simulink model "sst_three_phase_dab_three_levels_inv"  (R2025b)
settings: Solver=ode23tb  StartTime=0.0  StopTime=simlength  FixedStep=tc  MaxStep=tc
values from neighbouring files (symbols this model uses):
  Adrso = eye(2) + Arso*ts_inv    [init_model.m]
  Aresd_max = eye(2) + Ares_max*ts_afe    [init_model.m]
  Aresd_min = eye(2) + Ares_min*ts_afe    [init_model.m]
  Aresd_nom = eye(2) + Ares_nom*ts_afe    [init_model.m]
  Bresd = Bres*ts_afe    [init_model.m]
  CFi_dc2 = 900e-6*4    (= 0.0036)    [init_model.m]
  Cresd = Cres    [init_model.m]
  Crso = [1 0]    [init_model.m]
  delta = 0.025    [init_model.m]
  freq = 50    [init_model.m]
  Iac_FS = I_phase_normalization_factor    [init_model.m]
  Idc_FS = max(Idab1_dc_nom,Idab2_dc_nom) * margin_factor    [init_model.m]
  iph_grid_pu_ref = 3.75    [init_model.m]
  ki_afe = 18    [init_model.m]
  ki_pll = 3140    [init_model.m]
  ki_rpi = 18    [init_model.m]
  kp_afe = 0.25    [init_model.m]
  kp_pll = 314    [init_model.m]
  kp_rpi = 0.25    [init_model.m]
  Ldrso = acker(Adrso',Crso',polesdrso)'    [init_model.m]
  LFu1_AFE = 0.33e-3    (= 0.00033)    [init_model.m]
  n_modules = 2    [init_model.m]
  RLFu1_AFE = 157*0.05*LFu1_AFE    (= 0.0025905)    [init_model.m]
  tc = ts_dab/1000*24    (= 1e-06)    [init_model.m]
  ts_afe = 1/fPWM_AFE    (= 0.00025)    [init_model.m]
  ts_inv = 1/fPWM_INV    (= 0.00025)    [init_model.m]
  Vac_FS = V_phase_normalization_factor    [init_model.m]
  Vdab2_dc_nom = 1500    [init_model.m]
  Vdc_FS = max(Vdab1_dc_nom,Vdab2_dc_nom) * margin_factor    [init_model.m]
undefined symbols (not defined in the file or in its folder): omega_grid_nom, V_phase_normalization_factor
libraries: fl_lib x80, nesl_utility x55, discrete_time_low_pass_filter x6, single_phase_transformer x6, pi_ctrl x4, three_phase_inverter_ideal_switch_based_model x4, three_phase_inverter_mosfet_based_with_thermal_model x4, single_phase_transformer_lib x3, three_phase_dab_modulator x2, dclink_for_three_levels x2, single_phase_three_levels_PWM_modulator x2, dq_vector_pi x2
(part 2 of 5)

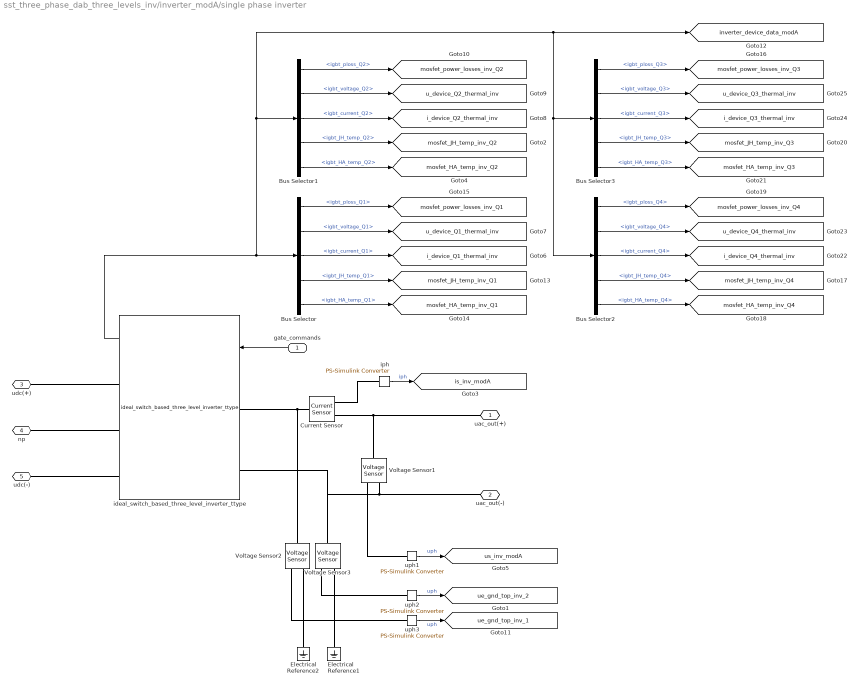
== system sst_three_phase_dab_three_levels_inv/inverter_modA/single phase inverter ==
  gate_commands : Inport
  Bus Selector : BusSelector  OutputSignals=igbt_ploss_Q1,igbt_voltage_Q1,igbt_current_Q1,igbt_JH_temp_Q1,igbt_HA_temp_Q1
  Bus Selector1 : BusSelector  OutputSignals=igbt_ploss_Q2,igbt_voltage_Q2,igbt_current_Q2,igbt_JH_temp_Q2,igbt_HA_temp_Q2
  Bus Selector2 : BusSelector  OutputSignals=igbt_ploss_Q4,igbt_voltage_Q4,igbt_current_Q4,igbt_JH_temp_Q4,igbt_HA_temp_Q4
  Bus Selector3 : BusSelector  OutputSignals=igbt_ploss_Q3,igbt_voltage_Q3,igbt_current_Q3,igbt_JH_temp_Q3,igbt_HA_temp_Q3
  Current Sensor : fl_lib/Electrical/Electrical Sensors/Current Sensor
  Electrical Reference1 : fl_lib/Electrical/Electrical Elements/Electrical Reference
  Electrical Reference2 : fl_lib/Electrical/Electrical Elements/Electrical Reference
  Voltage Sensor1 : fl_lib/Electrical/Electrical Sensors/Voltage Sensor
  Voltage Sensor2 : fl_lib/Electrical/Electrical Sensors/Voltage Sensor
  Voltage Sensor3 : fl_lib/Electrical/Electrical Sensors/Voltage Sensor
  ideal_switch_based_three_level_inverter_ttype : full_bridge_three_level_ttype_igbt_based_model/ideal_switch_based_three_level_inverter_ttype  Vth_inv_t=inv_t.Vth  Vce_sat_inv_t=inv_t.Vce_sat  Rce_on_inv_t=inv_t.Rce_on  Eon_inv_t=inv_t.Eon  Eoff_inv_t=inv_t.Eoff  Erec_inv_t=inv_t.Erec  Ion_sw_loss_inv_t=inv_t.Ion_sw_losses  Voff_sw_loss_inv_t=inv_t.Voff_sw_losses  Vdon_diode_inv_t=inv_t.Vdon_diode  Rdon_diode_inv_t=inv_t.Rdon_diode  rth_mosfet_JH_inv_t=inv_t.Rth_switch_JH  rth_mosfet_HA_inv_t=Rth_switch_HA  Csnubber_inv_t=inv_t.Csnubber  Rsnubber_inv_t=inv_t.Rsnubber  Vth_inv=inv.Vth  Vce_sat_inv=inv.Vce_sat  Rce_on_inv=inv.Rce_on  Eon_inv=inv.Eon  Eoff_inv=inv.Eoff  Erec_inv=inv.Erec  Ion_sw_loss_inv=inv.Ion_sw_losses  Voff_sw_loss_inv=inv.Voff_sw_losses  Vdon_diode_inv=inv.Vdon_diode  Rdon_diode_inv=inv.Rdon_diode  rth_mosfet_JH_inv=inv.Rth_switch_JH  rth_mosfet_HA_inv=Rth_mosfet_HA  Csnubber_inv=inv.Csnubber  Rsnubber_inv=inv.Rsnubber  tc=tc  JunctionTermalMass=JunctionTermalMass  mass_heatsink=weigth  specific_heat=cp_al  Tambient=Tambient  DThs_init=DThs_init
  iph : nesl_utility/PS-Simulink Converter  PhysicalDomain=network_engine_domain  SubClassName=ps_output  LeftPortType=input  RightPortType=output  PseudoPeriodic=off  Frequencies=[]  VectorFormat=1-D array  Unit=A  AffineConversion=off
  uph1 : nesl_utility/PS-Simulink Converter  PhysicalDomain=network_engine_domain  SubClassName=ps_output  LeftPortType=input  RightPortType=output  PseudoPeriodic=off  Frequencies=[]  VectorFormat=1-D array  Unit=V  AffineConversion=off
  uph2 : nesl_utility/PS-Simulink Converter  PhysicalDomain=network_engine_domain  SubClassName=ps_output  LeftPortType=input  RightPortType=output  PseudoPeriodic=off  Frequencies=[]  VectorFormat=1-D array  Unit=V  AffineConversion=off
  uph3 : nesl_utility/PS-Simulink Converter  PhysicalDomain=network_engine_domain  SubClassName=ps_output  LeftPortType=input  RightPortType=output  PseudoPeriodic=off  Frequencies=[]  VectorFormat=1-D array  Unit=V  AffineConversion=off
  uac_out(+) : PMIOPort  Side=Left
  uac_out(-) : PMIOPort  Port=2  Side=Left
  udc(+) : PMIOPort  Port=3  Side=Right
  np : PMIOPort  Port=4  Side=Right
  udc(-) : PMIOPort  Port=5  Side=Right
  tag scope: i_device_Q1_thermal_inv=global, i_device_Q2_thermal_inv=global, i_device_Q3_thermal_inv=global, i_device_Q4_thermal_inv=global, inverter_device_data_modA=global, is_inv_modA=global, mosfet_HA_temp_inv_Q1=global, mosfet_HA_temp_inv_Q2=global, mosfet_HA_temp_inv_Q3=global, mosfet_HA_temp_inv_Q4=global, mosfet_JH_temp_inv_Q1=global, mosfet_JH_temp_inv_Q2=global, mosfet_JH_temp_inv_Q3=global, mosfet_JH_temp_inv_Q4=global, mosfet_power_losses_inv_Q1=global, mosfet_power_losses_inv_Q2=global, mosfet_power_losses_inv_Q3=global, mosfet_power_losses_inv_Q4=global, u_device_Q1_thermal_inv=global, u_device_Q2_thermal_inv=global, u_device_Q3_thermal_inv=global, u_device_Q4_thermal_inv=global, ue_gnd_top_inv_1=global, ue_gnd_top_inv_2=global, us_inv_modA=global
  wires:
  iph/1 -> [is_inv_modA]  "iph"
  uph1/1 -> [us_inv_modA]  "uph"
  gate_commands/1 -> ideal_switch_based_three_level_inverter_ttype/1
  Bus Selector/1 -> [mosfet_power_losses_inv_Q1]  "<igbt_ploss_Q1>"
  Bus Selector/2 -> [u_device_Q1_thermal_inv]  "<igbt_voltage_Q1>"
  Bus Selector/3 -> [i_device_Q1_thermal_inv]  "<igbt_current_Q1>"
  Bus Selector/4 -> [mosfet_JH_temp_inv_Q1]  "<igbt_JH_temp_Q1>"
  Bus Selector/5 -> [mosfet_HA_temp_inv_Q1]  "<igbt_HA_temp_Q1>"
  Bus Selector1/4 -> [mosfet_JH_temp_inv_Q2]  "<igbt_JH_temp_Q2>"
  Bus Selector1/5 -> [mosfet_HA_temp_inv_Q2]  "<igbt_HA_temp_Q2>"
  Bus Selector1/3 -> [i_device_Q2_thermal_inv]  "<igbt_current_Q2>"
  Bus Selector1/2 -> [u_device_Q2_thermal_inv]  "<igbt_voltage_Q2>"
  Bus Selector1/1 -> [mosfet_power_losses_inv_Q2]  "<igbt_ploss_Q2>"
  uph2/1 -> [ue_gnd_top_inv_2]  "uph"
  uph3/1 -> [ue_gnd_top_inv_1]  "uph"
  ideal_switch_based_three_level_inverter_ttype/1 -> Bus Selector2/1, Bus Selector3/1, [inverter_device_data_modA], Bus Selector1/1, Bus Selector/1
  Bus Selector3/1 -> [mosfet_power_losses_inv_Q3]  "<igbt_ploss_Q3>"
  Bus Selector3/2 -> [u_device_Q3_thermal_inv]  "<igbt_voltage_Q3>"
  Bus Selector3/3 -> [i_device_Q3_thermal_inv]  "<igbt_current_Q3>"
  Bus Selector3/5 -> [mosfet_HA_temp_inv_Q3]  "<igbt_HA_temp_Q3>"
  Bus Selector3/4 -> [mosfet_JH_temp_inv_Q3]  "<igbt_JH_temp_Q3>"
  Bus Selector2/5 -> [mosfet_HA_temp_inv_Q4]  "<igbt_HA_temp_Q4>"
  Bus Selector2/4 -> [mosfet_JH_temp_inv_Q4]  "<igbt_JH_temp_Q4>"
  Bus Selector2/3 -> [i_device_Q4_thermal_inv]  "<igbt_current_Q4>"
  Bus Selector2/2 -> [u_device_Q4_thermal_inv]  "<igbt_voltage_Q4>"
  Bus Selector2/1 -> [mosfet_power_losses_inv_Q4]  "<igbt_ploss_Q4>"
  connections:
  Current Sensor/RConn1 -- iph/LConn1
  Current Sensor/RConn2 -- Voltage Sensor1/LConn1 -- uac_out(+)/RConn1
  Voltage Sensor1/RConn1 -- uph1/LConn1
  Voltage Sensor1/RConn2 -- ideal_switch_based_three_level_inverter_ttype/LConn2 -- Voltage Sensor3/LConn1 -- uac_out(-)/RConn1
  ideal_switch_based_three_level_inverter_ttype/RConn1 -- udc(+)/RConn1
  Current Sensor/LConn1 -- ideal_switch_based_three_level_inverter_ttype/LConn1 -- Voltage Sensor2/LConn1
  ideal_switch_based_three_level_inverter_ttype/RConn3 -- udc(-)/RConn1
  Electrical Reference2/LConn1 -- Voltage Sensor2/RConn2
  Electrical Reference1/LConn1 -- Voltage Sensor3/RConn2
  uph2/LConn1 -- Voltage Sensor3/RConn1
  uph3/LConn1 -- Voltage Sensor2/RConn1
  np/RConn1 -- ideal_switch_based_three_level_inverter_ttype/RConn2

== system sst_three_phase_dab_three_levels_inv/inverter_modA/single phase inverter control1 ==
  Constant : Constant
  acquisition_and_scaling_current : Subsystem
  acquisition_and_scaling_dc_voltage : Subsystem
  acquisition_and_scaling_voltage : Subsystem
  acquisition_and_scaling_voltage1 : Subsystem
  inverter_current_output_pu_reference : Subsystem
  pwm modulator : Subsystem
  rpi_based_single_phase_inverter_ctrl : Subsystem
  gate_cmds : Outport
  u_ctrl_out : Outport  Port=2
  tag scope: phase_synch_modA=global
  wires:
  [is_inv_modA] -> acquisition_and_scaling_current/1(in)
  pwm modulator/1(gate_cmds) -> gate_cmds/1
  [TRGO_INV_1] -> rpi_based_single_phase_inverter_ctrl/Trigger
  [inverter_voltage_output_modA] -> acquisition_and_scaling_voltage/1(in)
  acquisition_and_scaling_current/1(out) -> rpi_based_single_phase_inverter_ctrl/2(is_inv_pu)  "is_inv_pu"
  acquisition_and_scaling_voltage/1(out) -> rpi_based_single_phase_inverter_ctrl/1(inverter_voltage_output_pu)  "inverter_voltage_output_pu"
  inverter_current_output_pu_reference/1(inverter_current_output_pu_reference) -> rpi_based_single_phase_inverter_ctrl/3(is_inv_pu_reference)  "inverter_current_output_pu_reference"
  [dclink_voltage_inverter_modA] -> acquisition_and_scaling_dc_voltage/1(in)
  rpi_based_single_phase_inverter_ctrl/1(u_ctrl_out) -> u_ctrl_out/1, pwm modulator/1(vout)
  acquisition_and_scaling_voltage1/1(out) -> rpi_based_single_phase_inverter_ctrl/5(u_line_pu)  "ac_grid_voltage_pu"
  [ac_grid_voltage] -> acquisition_and_scaling_voltage1/1(in)
  rpi_based_single_phase_inverter_ctrl/2(phase_grid_modA) -> [phase_synch_modA]
  Constant/1 -> rpi_based_single_phase_inverter_ctrl/4(dclink_voltage_pu)
  [time_afe_module_1] -> rpi_based_single_phase_inverter_ctrl/6(time_afe_module_1)  "time_afe_module_1"

== system sst_three_phase_dab_three_levels_inv/inverter_modB/single phase inverter ==
  gate_commands : Inport
  Bus Selector : BusSelector  OutputSignals=switch_voltage_Q1,switch_current_Q1
  Current Sensor : fl_lib/Electrical/Electrical Sensors/Current Sensor
  Electrical Reference1 : fl_lib/Electrical/Electrical Elements/Electrical Reference
  Electrical Reference2 : fl_lib/Electrical/Electrical Elements/Electrical Reference
  Voltage Sensor1 : fl_lib/Electrical/Electrical Sensors/Voltage Sensor
  Voltage Sensor2 : fl_lib/Electrical/Electrical Sensors/Voltage Sensor
  Voltage Sensor3 : fl_lib/Electrical/Electrical Sensors/Voltage Sensor
  ideal_switch_based_three_level_inverter_ttype : full_bridge_three_level_ttype_ideal_switch_based_model/ideal_switch_based_three_level_inverter_ttype  Vth=5.5  Ron=1.5e-3  Vdon_diode=2  Rdon_diode=0.15e-3  Csnubber=10e-9  Rsnubber=2200
  iph : nesl_utility/PS-Simulink Converter  PhysicalDomain=network_engine_domain  SubClassName=ps_output  LeftPortType=input  RightPortType=output  PseudoPeriodic=off  Frequencies=[]  VectorFormat=1-D array  Unit=A  AffineConversion=off
  uph1 : nesl_utility/PS-Simulink Converter  PhysicalDomain=network_engine_domain  SubClassName=ps_output  LeftPortType=input  RightPortType=output  PseudoPeriodic=off  Frequencies=[]  VectorFormat=1-D array  Unit=V  AffineConversion=off
  uph2 : nesl_utility/PS-Simulink Converter  PhysicalDomain=network_engine_domain  SubClassName=ps_output  LeftPortType=input  RightPortType=output  PseudoPeriodic=off  Frequencies=[]  VectorFormat=1-D array  Unit=V  AffineConversion=off
  uph3 : nesl_utility/PS-Simulink Converter  PhysicalDomain=network_engine_domain  SubClassName=ps_output  LeftPortType=input  RightPortType=output  PseudoPeriodic=off  Frequencies=[]  VectorFormat=1-D array  Unit=V  AffineConversion=off
  uac_out(+) : PMIOPort  Side=Left
  uac_out(-) : PMIOPort  Port=2  Side=Left
  udc(+) : PMIOPort  Port=3  Side=Right
  np : PMIOPort  Port=4  Side=Right
  udc(-) : PMIOPort  Port=5  Side=Right
  tag scope: i_device_Q1_ideal_inv_modB=global, inverter_device_data_modB=global, is_inv_modB=global, u_device_Q1_ideal_inv_modB=global, ue_gnd_bottom_inv_1=global, ue_gnd_bottom_inv_2=global, us_inv_modB=global
  wires:
  gate_commands/1 -> ideal_switch_based_three_level_inverter_ttype/1
  uph1/1 -> [us_inv_modB]  "uph"
  iph/1 -> [is_inv_modB]  "iph"
  uph3/1 -> [ue_gnd_bottom_inv_1]  "uph"
  uph2/1 -> [ue_gnd_bottom_inv_2]  "uph"
  ideal_switch_based_three_level_inverter_ttype/1 -> [inverter_device_data_modB], Bus Selector/1
  Bus Selector/2 -> [i_device_Q1_ideal_inv_modB]  "<switch_current_Q1>"
  Bus Selector/1 -> [u_device_Q1_ideal_inv_modB]  "<switch_voltage_Q1>"
  connections:
  ideal_switch_based_three_level_inverter_ttype/RConn3 -- udc(-)/RConn1
  Voltage Sensor2/LConn1 -- ideal_switch_based_three_level_inverter_ttype/LConn1 -- Current Sensor/LConn1
  ideal_switch_based_three_level_inverter_ttype/RConn1 -- udc(+)/RConn1
  uac_out(-)/RConn1 -- ideal_switch_based_three_level_inverter_ttype/LConn2 -- Voltage Sensor3/LConn1 -- Voltage Sensor1/RConn2
  Voltage Sensor1/RConn1 -- uph1/LConn1
  uac_out(+)/RConn1 -- Voltage Sensor1/LConn1 -- Current Sensor/RConn2
  Current Sensor/RConn1 -- iph/LConn1
  Electrical Reference2/LConn1 -- Voltage Sensor2/RConn2
  uph2/LConn1 -- Voltage Sensor3/RConn1
  uph3/LConn1 -- Voltage Sensor2/RConn1
  Electrical Reference1/LConn1 -- Voltage Sensor3/RConn2
  np/RConn1 -- ideal_switch_based_three_level_inverter_ttype/RConn2

== system sst_three_phase_dab_three_levels_inv/inverter_modB/single phase inverter control1 ==
  Constant : Constant
  acquisition_and_scaling_current : Subsystem
  acquisition_and_scaling_dc_voltage : Subsystem
  acquisition_and_scaling_voltage : Subsystem
  acquisition_and_scaling_voltage1 : Subsystem
  inverter_current_output_pu_reference : Subsystem
  pwm modulator : Subsystem
  rpi_based_single_phase_inverter_ctrl : Subsystem
  gate_cmds : Outport
  tag scope: phase_synch_modB=global
  wires:
  pwm modulator/1(gate_cmds) -> gate_cmds/1
  rpi_based_single_phase_inverter_ctrl/2(phase_grid_modA) -> [phase_synch_modB]
  rpi_based_single_phase_inverter_ctrl/1(u_ctrl_out) -> pwm modulator/1(vout)
  [u_ctrl_out_master] -> rpi_based_single_phase_inverter_ctrl/6(u_ctrl_out_master)  "u_ctrl_out_master"
  Constant/1 -> rpi_based_single_phase_inverter_ctrl/4(dclink_voltage_pu)
  acquisition_and_scaling_voltage1/1(out) -> rpi_based_single_phase_inverter_ctrl/5(u_line_pu)  "u_line_pu"
  acquisition_and_scaling_current/1(out) -> rpi_based_single_phase_inverter_ctrl/2(is_inv_pu)  "is_inv_pu"
  [inverter_voltage_output_modB] -> acquisition_and_scaling_voltage/1(in)
  [ac_grid_voltage] -> acquisition_and_scaling_voltage1/1(in)
  acquisition_and_scaling_voltage/1(out) -> rpi_based_single_phase_inverter_ctrl/1(inverter_voltage_output_pu)  "inverter_voltage_output_pu"
  [dclink_voltage_inverter_modB] -> acquisition_and_scaling_dc_voltage/1(in)
  [is_inv_modB] -> acquisition_and_scaling_current/1(in)
  inverter_current_output_pu_reference/1(inverter_current_output_pu_reference) -> rpi_based_single_phase_inverter_ctrl/3(is_inv_pu_reference)  "inverter_current_output_pu_reference"
  [TRGO_INV_2] -> rpi_based_single_phase_inverter_ctrl/Trigger

== system sst_three_phase_dab_three_levels_inv/line_source/phase_gen ==
  Constant4 : Constant  Value=50*2*pi
  Integrator : Integrator
  bounder1 : MATLAB Function  TreatAsAtomicUnit=on
  phase_gen : Outport  VectorParamsAs1DForOutWhenUnconnected=off
  wires:
  Constant4/1 -> Integrator/1
  Integrator/1 -> bounder1/1(u)
  bounder1/1(y) -> phase_gen/1  "grid_emu_phase"

== system sst_three_phase_dab_three_levels_inv/scopes/scopes_dab_modA ==
  Bus Selector : BusSelector  OutputSignals=mosfet_ploss_Q1,mosfet_ploss_Q2
  Bus Selector1 : BusSelector  OutputSignals=mosfet_ploss_Q1,mosfet_ploss_Q2
  dab TR i2/i1 modA : Scope  NumInputPorts=2
      settings: SampleTime=tc  ActiveDisplayYMinimum=-1515.8601129634949  ActiveDisplayYMaximum=1519.4045908602914  DataLoggingVariableName=ScopeData13
  dab TR u2/u1 modA : Scope  NumInputPorts=2
      settings: SampleTime=tc  ActiveDisplayYMinimum=-893.62031856834165  ActiveDisplayYMaximum=653.92363611228757  DataLoggingVariableName=ScopeData4
  dab current output/input modA : Scope  NumInputPorts=2
      settings: SampleTime=tc  ActiveDisplayYMinimum=-34.407086049322743  ActiveDisplayYMaximum=284.20809963586862  DataLoggingVariableName=ScopeData8
  dab outputs modA : Scope  NumInputPorts=2
      settings: SampleTime=tc  ActiveDisplayYMinimum=-1504.2584903012705  ActiveDisplayYMaximum=905.23681286440785  DataLoggingVariableName=ScopeData6
  dab voltage input/output modA : Scope  NumInputPorts=2
      settings: SampleTime=tc  ActiveDisplayYMinimum=-224.45374462345234  ActiveDisplayYMaximum=1977.0471198962268  DataLoggingVariableName=ScopeData10
  dab_analysis_modA : Scope  NumInputPorts=4
      settings: SampleTime=tc  ActiveDisplayYMinimum=-2404.4721774395748  ActiveDisplayYMaximum=2406.0057347567245  DataLoggingVariableName=ScopeData15
  dab_analysis_power loss : Scope  NumInputPorts=4
      settings: SampleTime=tc  ActiveDisplayYMinimum=-34.96618025113866  ActiveDisplayYMaximum=361.139187884934  DataLoggingVariableName=ScopeData17
  wires:
  [dab_voltage_input_modA] -> dab voltage input/output modA/1  "dab_voltage_input_modA"
  [dab_current_output_modA] -> dab current output/input modA/1  "dab_current_output_modA"
  [dab_voltage_output_modA] -> dab voltage input/output modA/2  "dab_voltage_output_modA"
  [dab_current_input_modA] -> dab current output/input modA/2  "dab_current_input_modA"
  [i2_dab_transformer_modA] -> dab TR i2/i1 modA/1  "i2_dab_transformer_modA"
  [i1_dab_transformer_modA] -> dab TR i2/i1 modA/2  "i1_dab_transformer_modA"
  [u2_dab_transformer_modA] -> dab TR u2/u1 modA/1  "u2_dab_transformer_modA"
  [u1_dab_transformer_modA] -> dab TR u2/u1 modA/2  "u1_dab_transformer_modA"
  [dab_voltage_output_modA] -> dab outputs modA/2  "dab_voltage_output_modA"
  [dab_current_output_modA] -> dab outputs modA/1  "dab_current_output_modA"
  [i2_dab_transformer_modA] -> dab_analysis_modA/1  "i2_dab_transformer_modA"
  [i1_dab_transformer_modA] -> dab_analysis_modA/2  "i1_dab_transformer_modA"
  [u1_dab_transformer_modA] -> dab_analysis_modA/3  "u1_dab_transformer_modA"
  [u2_dab_transformer_modA] -> dab_analysis_modA/4  "u2_dab_transformer_modA"
  [inverter_1_dab_devices_modA] -> Bus Selector/1
  [inverter_2_dab_devices_modA] -> Bus Selector1/1
  Bus Selector/1 -> dab_analysis_power loss/1  "<mosfet_ploss_Q1>"
  Bus Selector/2 -> dab_analysis_power loss/2  "<mosfet_ploss_Q2>"
  Bus Selector1/1 -> dab_analysis_power loss/3  "<mosfet_ploss_Q1>"
  Bus Selector1/2 -> dab_analysis_power loss/4  "<mosfet_ploss_Q2>"

== system sst_three_phase_dab_three_levels_inv/scopes/scopes_dab_modB ==
  dab TR i2/i1 modB : Scope  NumInputPorts=2
      settings: SampleTime=tc  ActiveDisplayYMinimum=-700.08630880673149  ActiveDisplayYMaximum=469.74027472719069  DataLoggingVariableName=ScopeData13
  dab TR u2/u1 modB : Scope  NumInputPorts=2
      settings: SampleTime=tc  ActiveDisplayYMinimum=-893.62031856834165  ActiveDisplayYMaximum=653.92363611228757  DataLoggingVariableName=ScopeData4
  dab current output/input modB : Scope  NumInputPorts=2
      settings: SampleTime=tc  ActiveDisplayYMinimum=-7335.7913745283768  ActiveDisplayYMaximum=23819.434208451414  DataLoggingVariableName=ScopeData8
  dab outputs modB : Scope  NumInputPorts=2
      settings: SampleTime=tc  ActiveDisplayYMinimum=-1276.7812228163118  ActiveDisplayYMaximum=1202.3221787513703  DataLoggingVariableName=ScopeData6
  dab voltage input/output modB : Scope  NumInputPorts=2
      settings: SampleTime=tc  ActiveDisplayYMinimum=-237.60937353263552  ActiveDisplayYMaximum=2138.4843617937204  DataLoggingVariableName=ScopeData10
  dab_analysis_modB : Scope  NumInputPorts=4
      settings: SampleTime=tc  ActiveDisplayYMinimum=-1515.8601129634949  ActiveDisplayYMaximum=1519.4045908602914  DataLoggingVariableName=ScopeData15
  wires:
  [u2_dab_transformer_modB] -> dab_analysis_modB/4  "u2_dab_transformer_modB"
  [u1_dab_transformer_modB] -> dab_analysis_modB/3  "u1_dab_transformer_modB"
  [i1_dab_transformer_modB] -> dab_analysis_modB/2  "i1_dab_transformer_modB"
  [i2_dab_transformer_modB] -> dab_analysis_modB/1  "i2_dab_transformer_modB"
  [dab_current_output_modB] -> dab outputs modB/1  "dab_current_output_modB"
  [dab_voltage_output_modB] -> dab outputs modB/2  "dab_voltage_output_modB"
  [u1_dab_transformer_modB] -> dab TR u2/u1 modB/2  "u1_dab_transformer_modB"
  [u2_dab_transformer_modB] -> dab TR u2/u1 modB/1  "u2_dab_transformer_modB"
  [i1_dab_transformer_modB] -> dab TR i2/i1 modB/2  "i1_dab_transformer_modB"
  [i2_dab_transformer_modB] -> dab TR i2/i1 modB/1  "i2_dab_transformer_modB"
  [dab_current_input_modB] -> dab current output/input modB/2  "dab_current_input_modB"
  [dab_voltage_output_modB] -> dab voltage input/output modB/2  "dab_voltage_output_modB"
  [dab_current_output_modB] -> dab current output/input modB/1  "dab_current_output_modB"
  [dab_voltage_input_modB] -> dab voltage input/output modB/1  "dab_voltage_input_modB"

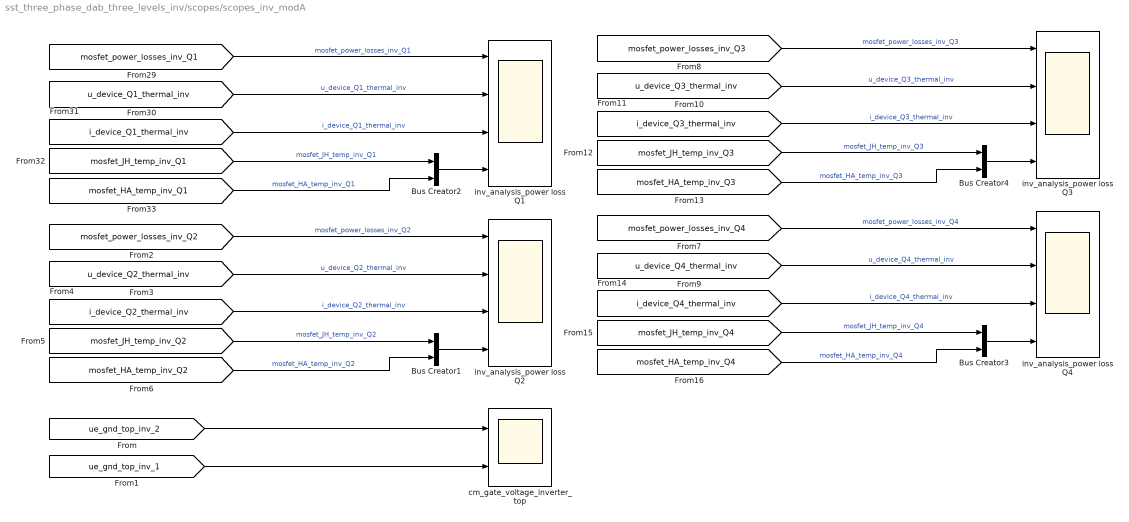
== system sst_three_phase_dab_three_levels_inv/scopes/scopes_inv_modA ==
  Bus Creator{1..4} (4 alike) : BusCreator  Inputs=2
  cm_gate_voltage_inverter_top : Scope  NumInputPorts=2
      settings: SampleTime=tc  ActiveDisplayYMinimum=-1089.6954299405313  ActiveDisplayYMaximum=1165.8713445946826  DataLoggingVariableName=ScopeData22
  inv_analysis_power loss Q{1..4} (4 alike) : Scope  NumInputPorts=4
      inv_analysis_power loss Q1 settings: SampleTime=tc  ActiveDisplayYMinimum=480.40088519857073  ActiveDisplayYMaximum=655.06729010423419  DataLoggingVariableName=ScopeData18
      inv_analysis_power loss Q2 settings: SampleTime=tc  ActiveDisplayYMinimum=-297.99280090077724  ActiveDisplayYMaximum=2682.0574560934515  DataLoggingVariableName=ScopeData5
      inv_analysis_power loss Q3 settings: SampleTime=tc  ActiveDisplayYMinimum=-300.61802767301606  ActiveDisplayYMaximum=3732.3996801361568  DataLoggingVariableName=ScopeData16
      inv_analysis_power loss Q4 settings: SampleTime=tc  ActiveDisplayYMinimum=-24.066330497867384  ActiveDisplayYMaximum=465.0901731737107  DataLoggingVariableName=ScopeData19
  wires:
  [mosfet_JH_temp_inv_Q1] -> Bus Creator2/1  "mosfet_JH_temp_inv_Q1"
  [u_device_Q1_thermal_inv] -> inv_analysis_power loss Q1/2  "u_device_Q1_thermal_inv"
  [i_device_Q1_thermal_inv] -> inv_analysis_power loss Q1/3  "i_device_Q1_thermal_inv"
  [mosfet_HA_temp_inv_Q1] -> Bus Creator2/2  "mosfet_HA_temp_inv_Q1"
  Bus Creator2/1 -> inv_analysis_power loss Q1/4
  [mosfet_power_losses_inv_Q1] -> inv_analysis_power loss Q1/1  "mosfet_power_losses_inv_Q1"
  [ue_gnd_top_inv_2] -> cm_gate_voltage_inverter_top/1
  [ue_gnd_top_inv_1] -> cm_gate_voltage_inverter_top/2
  [mosfet_power_losses_inv_Q2] -> inv_analysis_power loss Q2/1  "mosfet_power_losses_inv_Q2"
  Bus Creator1/1 -> inv_analysis_power loss Q2/4
  [mosfet_HA_temp_inv_Q2] -> Bus Creator1/2  "mosfet_HA_temp_inv_Q2"
  [i_device_Q2_thermal_inv] -> inv_analysis_power loss Q2/3  "i_device_Q2_thermal_inv"
  [u_device_Q2_thermal_inv] -> inv_analysis_power loss Q2/2  "u_device_Q2_thermal_inv"
  [mosfet_JH_temp_inv_Q2] -> Bus Creator1/1  "mosfet_JH_temp_inv_Q2"
  [mosfet_JH_temp_inv_Q4] -> Bus Creator3/1  "mosfet_JH_temp_inv_Q4"
  [u_device_Q4_thermal_inv] -> inv_analysis_power loss Q4/2  "u_device_Q4_thermal_inv"
  [i_device_Q4_thermal_inv] -> inv_analysis_power loss Q4/3  "i_device_Q4_thermal_inv"
  [mosfet_HA_temp_inv_Q4] -> Bus Creator3/2  "mosfet_HA_temp_inv_Q4"
  Bus Creator3/1 -> inv_analysis_power loss Q4/4
  [mosfet_power_losses_inv_Q4] -> inv_analysis_power loss Q4/1  "mosfet_power_losses_inv_Q4"
  [mosfet_power_losses_inv_Q3] -> inv_analysis_power loss Q3/1  "mosfet_power_losses_inv_Q3"
  Bus Creator4/1 -> inv_analysis_power loss Q3/4
  [mosfet_HA_temp_inv_Q3] -> Bus Creator4/2  "mosfet_HA_temp_inv_Q3"
  [i_device_Q3_thermal_inv] -> inv_analysis_power loss Q3/3  "i_device_Q3_thermal_inv"
  [u_device_Q3_thermal_inv] -> inv_analysis_power loss Q3/2  "u_device_Q3_thermal_inv"
  [mosfet_JH_temp_inv_Q3] -> Bus Creator4/1  "mosfet_JH_temp_inv_Q3"

== system sst_three_phase_dab_three_levels_inv/scopes/scopes_inv_modB ==
  cm_gate_voltage_inverter_bottom : Scope  NumInputPorts=2
      settings: SampleTime=tc  ActiveDisplayYMinimum=-1241.6958905586757  ActiveDisplayYMaximum=1224.9152234663466  DataLoggingVariableName=ScopeData22
  device_voltage_current_inv Q1 modB : Scope  NumInputPorts=3
      settings: SampleTime=tc  ActiveDisplayYMinimum=-236.24076950985182  ActiveDisplayYMaximum=2105.4029656396665  DataLoggingVariableName=ScopeData20
  wires:
  [ue_gnd_bottom_inv_1] -> cm_gate_voltage_inverter_bottom/2
  [ue_gnd_bottom_inv_2] -> cm_gate_voltage_inverter_bottom/1
  [i_device_Q1_ideal_inv_modB] -> device_voltage_current_inv Q1 modB/2  "iQ1"
  [u_device_Q1_ideal_inv_modB] -> device_voltage_current_inv Q1 modB/1  "uQ1"
  [udc12_inverter_modB] -> device_voltage_current_inv Q1 modB/3  "udcs"

== system sst_three_phase_dab_three_levels_inv/dab_modA/dab_ctrl/references ==
  Rate Limiter : RateLimiter  RisingSlewLimit=Vdab2_dc_nom*10  FallingSlewLimit=-Vdab2_dc_nom*10  SampleTimeMode=inherited
  Vout_dc_nom : Step  Time=1e-3  After=Vdab2_dc_nom  SampleTime=0
  vout_ref : Outport
  wires:
  Rate Limiter/1 -> vout_ref/1
  Vout_dc_nom/1 -> Rate Limiter/1

== system sst_three_phase_dab_three_levels_inv/dab_modA/dab_ctrl/sampling_i_filter1 ==
  in : Inport
  1/Ti3 : Gain  Gain=1/Idc_FS  OutDataTypeStr=double  SaturateOnIntegerOverflow=on  ParamDataTypeStr=Inherit: Same as input
  out_pu : Outport
  wires:
  in/1 -> 1/Ti3/1
  1/Ti3/1 -> out_pu/1

== system sst_three_phase_dab_three_levels_inv/dab_modA/dab_ctrl/sampling_v_filter1 ==
  in : Inport
  1/Ti3 : Gain  Gain=1/Vdc_FS  OutDataTypeStr=double  SaturateOnIntegerOverflow=on  ParamDataTypeStr=Inherit: Same as input
  out_pu : Outport
  wires:
  in/1 -> 1/Ti3/1
  1/Ti3/1 -> out_pu/1

== system sst_three_phase_dab_three_levels_inv/dab_modA/dab_ctrl/sampling_v_filter2 ==
  in : Inport
  1/Ti3 : Gain  Gain=1/Vdc_FS  OutDataTypeStr=double  SaturateOnIntegerOverflow=on  ParamDataTypeStr=Inherit: Same as input
  Saturation : Saturate  UpperLimit=1  LowerLimit=0  OutDataTypeStr=double
  out_pu : Outport
  wires:
  in/1 -> 1/Ti3/1
  1/Ti3/1 -> Saturation/1
  Saturation/1 -> out_pu/1

== system sst_three_phase_dab_three_levels_inv/dab_modA/dab_ctrl/ui_ctrl ==
  i_pu_dab_input : Inport
  u_pu_dab_output : Inport  Port=2
  u_pu_dab_output_ref : Inport  Port=3
  local_time_dab : Inport  Port=4
  Trigger : TriggerPort  VariantControl=(inherit)  PortDimensions=1
  Goto Tag Visibility : GotoTagVisibility  GotoTag=local_time
  Goto Tag Visibility1 : GotoTagVisibility  GotoTag=i_ctrl_out_dab
  Goto Tag Visibility2 : GotoTagVisibility  GotoTag=i_in_pu_dab
  Goto Tag Visibility3 : GotoTagVisibility  GotoTag=u_ctrl_out_dab
  Goto Tag Visibility4 : GotoTagVisibility  GotoTag=uout_ref_pu_dab
  Goto Tag Visibility5 : GotoTagVisibility  GotoTag=uout_pu_dab
  dab_ctrl : Subsystem
  scopes : Subsystem
  storage_data : Subsystem
  phase_displacement : Outport
  tag scope: local_time=scoped
  wires:
  i_pu_dab_input/1 -> dab_ctrl/1(i_pu_dab_input)
  u_pu_dab_output/1 -> dab_ctrl/2(u_pu_dab_output)
  u_pu_dab_output_ref/1 -> dab_ctrl/3(u_pu_dab_output_ref)
  dab_ctrl/1(phase_displacement) -> phase_displacement/1
  local_time_dab/1 -> [local_time]

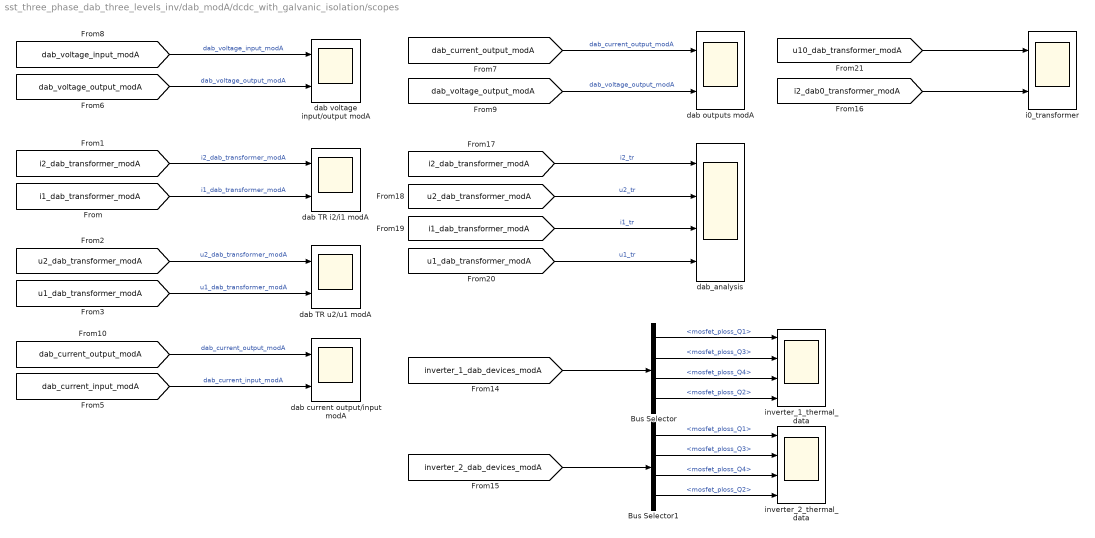
== system sst_three_phase_dab_three_levels_inv/dab_modA/dcdc_with_galvanic_isolation/scopes ==
  Bus Selector : BusSelector  OutputSignals=mosfet_ploss_Q1,mosfet_ploss_Q3,mosfet_ploss_Q4,mosfet_ploss_Q2
  Bus Selector1 : BusSelector  OutputSignals=mosfet_ploss_Q1,mosfet_ploss_Q3,mosfet_ploss_Q4,mosfet_ploss_Q2
  dab TR i2/i1 modA : Scope  NumInputPorts=2
      settings: SampleTime=tc  ActiveDisplayYMinimum=-769.76570927697639  ActiveDisplayYMaximum=617.34679539784429  DataLoggingVariableName=ScopeData13
  dab TR u2/u1 modA : Scope  NumInputPorts=2
      settings: SampleTime=tc  ActiveDisplayYMinimum=-1578.7453878307324  ActiveDisplayYMaximum=1578.7340154658184  DataLoggingVariableName=ScopeData4
  dab current output/input modA : Scope  NumInputPorts=2
      settings: SampleTime=tc  ActiveDisplayYMinimum=-410.50779379600635  ActiveDisplayYMaximum=588.57119970360964  DataLoggingVariableName=ScopeData8
  dab outputs modA : Scope  NumInputPorts=2
      settings: SampleTime=tc  ActiveDisplayYMinimum=-911.87281827356537  ActiveDisplayYMaximum=678.26507696890121  DataLoggingVariableName=ScopeData6
  dab voltage input/output modA : Scope  NumInputPorts=2
      settings: SampleTime=tc  ActiveDisplayYMinimum=1151.9301233458582  ActiveDisplayYMaximum=1294.7889710686802  DataLoggingVariableName=ScopeData10
  dab_analysis : Scope  NumInputPorts=4
      settings: SampleTime=tc  ActiveDisplayYMinimum=-2819.8939411691067  ActiveDisplayYMaximum=1653.00985583068  DataLoggingVariableName=ScopeData14
  i0_transformer : Scope  NumInputPorts=2
      settings: SampleTime=tc  ActiveDisplayYMinimum=-1.8947806286936003E-13  ActiveDisplayYMaximum=1.8947806286936003E-13  DataLoggingVariableName=ScopeData11
  inverter_1_thermal_data : Scope  NumInputPorts=4
      settings: SampleTime=tc  ActiveDisplayYMinimum=-41.628226428892724  ActiveDisplayYMaximum=374.65403786003458
  inverter_2_thermal_data : Scope  NumInputPorts=4
      settings: SampleTime=tc  ActiveDisplayYMinimum=-51.964921296072347  ActiveDisplayYMaximum=467.68429166465125  DataLoggingVariableName=ScopeData9
  wires:
  [dab_voltage_input_modA] -> dab voltage input/output modA/1  "dab_voltage_input_modA"
  [dab_current_output_modA] -> dab current output/input modA/1  "dab_current_output_modA"
  [dab_voltage_output_modA] -> dab voltage input/output modA/2  "dab_voltage_output_modA"
  [dab_current_input_modA] -> dab current output/input modA/2  "dab_current_input_modA"
  [i2_dab_transformer_modA] -> dab TR i2/i1 modA/1  "i2_dab_transformer_modA"
  [i1_dab_transformer_modA] -> dab TR i2/i1 modA/2  "i1_dab_transformer_modA"
  [u2_dab_transformer_modA] -> dab TR u2/u1 modA/1  "u2_dab_transformer_modA"
  [u1_dab_transformer_modA] -> dab TR u2/u1 modA/2  "u1_dab_transformer_modA"
  [dab_voltage_output_modA] -> dab outputs modA/2  "dab_voltage_output_modA"
  [dab_current_output_modA] -> dab outputs modA/1  "dab_current_output_modA"
  [inverter_1_dab_devices_modA] -> Bus Selector/1
  Bus Selector/1 -> inverter_1_thermal_data/1  "<mosfet_ploss_Q1>"
  Bus Selector/2 -> inverter_1_thermal_data/2  "<mosfet_ploss_Q3>"
  Bus Selector/3 -> inverter_1_thermal_data/3  "<mosfet_ploss_Q4>"
  Bus Selector/4 -> inverter_1_thermal_data/4  "<mosfet_ploss_Q2>"
  Bus Selector1/4 -> inverter_2_thermal_data/4  "<mosfet_ploss_Q2>"
  Bus Selector1/3 -> inverter_2_thermal_data/3  "<mosfet_ploss_Q4>"
  Bus Selector1/2 -> inverter_2_thermal_data/2  "<mosfet_ploss_Q3>"
  Bus Selector1/1 -> inverter_2_thermal_data/1  "<mosfet_ploss_Q1>"
  [inverter_2_dab_devices_modA] -> Bus Selector1/1
  [i2_dab0_transformer_modA] -> i0_transformer/2
  [u10_dab_transformer_modA] -> i0_transformer/1
  [u2_dab_transformer_modA] -> dab_analysis/2  "u2_tr"
  [i2_dab_transformer_modA] -> dab_analysis/1  "i2_tr"
  [u1_dab_transformer_modA] -> dab_analysis/4  "u1_tr"
  [i1_dab_transformer_modA] -> dab_analysis/3  "i1_tr"

== system sst_three_phase_dab_three_levels_inv/dab_modA/dcdc_with_galvanic_isolation/single_phase_dab_transformer ==
  three_phase_hf_transformer : Subsystem
  three_phase_hf_transformer1 : Subsystem  Commented=on
  threephase_vi_measures_stack : Subsystem
  threephase_vi_measures_stack1 : Subsystem
  u1 : PMIOPort  Side=Left
  v1 : PMIOPort  Port=2  Side=Left
  w1 : PMIOPort  Port=3  Side=Left
  u2 : PMIOPort  Port=4  Side=Right
  v2 : PMIOPort  Port=5  Side=Right
  w2 : PMIOPort  Port=6  Side=Right
  connections:
  three_phase_hf_transformer/LConn1 -- threephase_vi_measures_stack/RConn1
  three_phase_hf_transformer/LConn2 -- threephase_vi_measures_stack/RConn2
  three_phase_hf_transformer/LConn3 -- threephase_vi_measures_stack/RConn3
  threephase_vi_measures_stack1/LConn1 -- three_phase_hf_transformer/RConn1
  threephase_vi_measures_stack1/LConn2 -- three_phase_hf_transformer/RConn2
  threephase_vi_measures_stack1/LConn3 -- three_phase_hf_transformer/RConn3
  threephase_vi_measures_stack1/LConn4 -- three_phase_hf_transformer/RConn4
  threephase_vi_measures_stack/RConn4 -- three_phase_hf_transformer/LConn4
  u1/RConn1 -- threephase_vi_measures_stack/LConn1
  v1/RConn1 -- threephase_vi_measures_stack/LConn2
  w1/RConn1 -- threephase_vi_measures_stack/LConn3
  v2/RConn1 -- threephase_vi_measures_stack1/RConn2
  w2/RConn1 -- threephase_vi_measures_stack1/RConn3
  threephase_vi_measures_stack1/RConn1 -- u2/RConn1

== system sst_three_phase_dab_three_levels_inv/dab_modA/dcdc_with_galvanic_isolation/three_phase_inverter_1 ==
  gate_commands : Inport
  dclink_1 : Subsystem
  three_phase_inverter_1 : Subsystem
  u : PMIOPort  Side=Left
  v : PMIOPort  Port=2  Side=Left
  Udc(+) : PMIOPort  Port=3  Side=Right
  Udc(-) : PMIOPort  Port=4  Side=Right
  w : PMIOPort  Port=5  Side=Left
  wires:
  gate_commands/1 -> three_phase_inverter_1/1(gate_commands)
  connections:
  Udc(+)/RConn1 -- dclink_1/LConn1
  Udc(-)/RConn1 -- dclink_1/LConn2
  dclink_1/RConn1 -- three_phase_inverter_1/LConn1
  three_phase_inverter_1/RConn1 -- u/RConn1
  three_phase_inverter_1/RConn2 -- v/RConn1
  three_phase_inverter_1/LConn2 -- dclink_1/RConn2
  w/RConn1 -- three_phase_inverter_1/RConn3

== system sst_three_phase_dab_three_levels_inv/dab_modA/dcdc_with_galvanic_isolation/three_phase_inverter_2 ==
  gate_commands : Inport
  dclink_2 : Subsystem
  three_phase_inverter_2 : Subsystem
  u : PMIOPort  Side=Left
  v : PMIOPort  Port=2  Side=Left
  udc(+) : PMIOPort  Port=3  Side=Right
  udc(-) : PMIOPort  Port=4  Side=Right
  w : PMIOPort  Port=5  Side=Left
  wires:
  gate_commands/1 -> three_phase_inverter_2/1(gate_commands)
  connections:
  udc(+)/RConn1 -- dclink_2/RConn1
  udc(-)/RConn1 -- dclink_2/RConn2
  dclink_2/LConn1 -- three_phase_inverter_2/RConn1
  u/RConn1 -- three_phase_inverter_2/LConn1
  v/RConn1 -- three_phase_inverter_2/LConn2
  dclink_2/LConn2 -- three_phase_inverter_2/RConn2
  w/RConn1 -- three_phase_inverter_2/LConn3

== system sst_three_phase_dab_three_levels_inv/dab_modB/dab_ctrl/references ==
  Rate Limiter : RateLimiter  RisingSlewLimit=Vdab2_dc_nom*10  FallingSlewLimit=-Vdab2_dc_nom*10  SampleTimeMode=inherited
  Vout_dc_nom : Step  Time=1e-3  After=Vdab2_dc_nom  SampleTime=0
  vout_ref : Outport
  wires:
  Vout_dc_nom/1 -> Rate Limiter/1
  Rate Limiter/1 -> vout_ref/1

== system sst_three_phase_dab_three_levels_inv/dab_modB/dab_ctrl/sampling_i_filter1 ==
  in : Inport
  1/Ti3 : Gain  Gain=1/Idc_FS  OutDataTypeStr=double  SaturateOnIntegerOverflow=on  ParamDataTypeStr=Inherit: Same as input
  out_pu : Outport
  wires:
  1/Ti3/1 -> out_pu/1
  in/1 -> 1/Ti3/1

== system sst_three_phase_dab_three_levels_inv/dab_modB/dab_ctrl/sampling_v_filter1 ==
  in : Inport
  1/Ti3 : Gain  Gain=1/Vdc_FS  OutDataTypeStr=double  SaturateOnIntegerOverflow=on  ParamDataTypeStr=Inherit: Same as input
  out_pu : Outport
  wires:
  1/Ti3/1 -> out_pu/1
  in/1 -> 1/Ti3/1

== system sst_three_phase_dab_three_levels_inv/dab_modB/dab_ctrl/sampling_v_filter2 ==
  in : Inport
  1/Ti3 : Gain  Gain=1/Vdc_FS  OutDataTypeStr=double  SaturateOnIntegerOverflow=on  ParamDataTypeStr=Inherit: Same as input
  Saturation : Saturate  UpperLimit=1  LowerLimit=0  OutDataTypeStr=double
  out_pu : Outport
  wires:
  Saturation/1 -> out_pu/1
  1/Ti3/1 -> Saturation/1
  in/1 -> 1/Ti3/1

== system sst_three_phase_dab_three_levels_inv/dab_modB/dab_ctrl/ui_ctrl ==
  i_pu_dab_input : Inport
  u_pu_dab_output : Inport  Port=2
  u_pu_dab_output_ref : Inport  Port=3
  local_time_dab : Inport  Port=4
  Trigger : TriggerPort  VariantControl=(inherit)  PortDimensions=1
  Goto Tag Visibility : GotoTagVisibility  GotoTag=local_time
  Goto Tag Visibility1 : GotoTagVisibility  GotoTag=i_ctrl_out_dab
  Goto Tag Visibility2 : GotoTagVisibility  GotoTag=i_in_pu_dab
  Goto Tag Visibility3 : GotoTagVisibility  GotoTag=u_ctrl_out_dab
  Goto Tag Visibility4 : GotoTagVisibility  GotoTag=uout_ref_pu_dab
  Goto Tag Visibility5 : GotoTagVisibility  GotoTag=uout_pu_dab
  dab_ctrl : Subsystem
  scopes : Subsystem
  storage_data : Subsystem
  phase_displacement : Outport
  tag scope: local_time=scoped
  wires:
  local_time_dab/1 -> [local_time]
  dab_ctrl/1(phase_displacement) -> phase_displacement/1
  u_pu_dab_output_ref/1 -> dab_ctrl/3(u_pu_dab_output_ref)
  u_pu_dab_output/1 -> dab_ctrl/2(u_pu_dab_output)
  i_pu_dab_input/1 -> dab_ctrl/1(i_pu_dab_input)

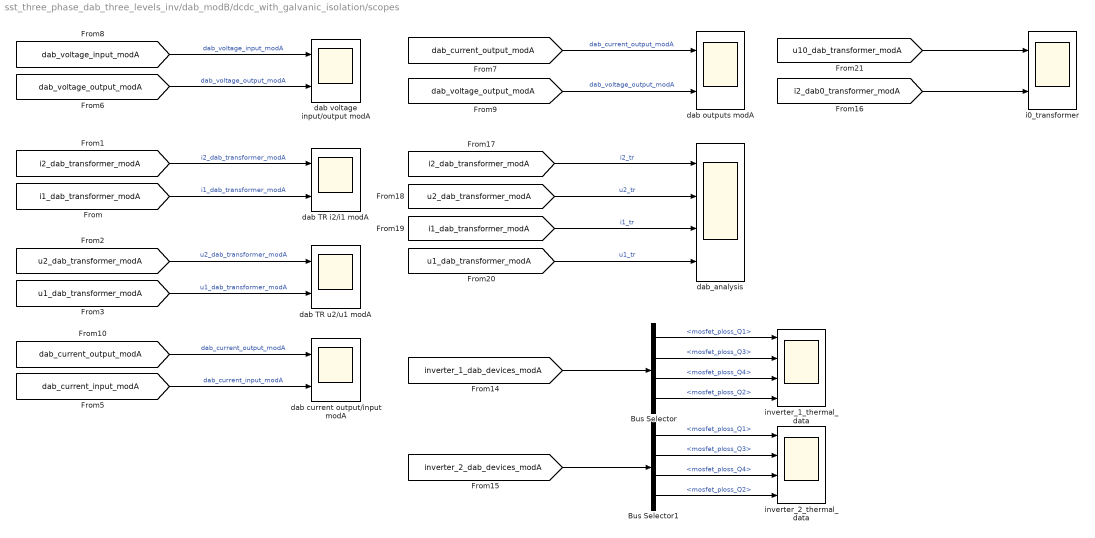
== system sst_three_phase_dab_three_levels_inv/dab_modB/dcdc_with_galvanic_isolation/scopes ==
  Bus Selector : BusSelector  OutputSignals=mosfet_ploss_Q1,mosfet_ploss_Q3,mosfet_ploss_Q4,mosfet_ploss_Q2
  Bus Selector1 : BusSelector  OutputSignals=mosfet_ploss_Q1,mosfet_ploss_Q3,mosfet_ploss_Q4,mosfet_ploss_Q2
  dab TR i2/i1 modA : Scope  NumInputPorts=2
      settings: SampleTime=tc  ActiveDisplayYMinimum=-769.76570927697639  ActiveDisplayYMaximum=617.34679539784429  DataLoggingVariableName=ScopeData13
  dab TR u2/u1 modA : Scope  NumInputPorts=2
      settings: SampleTime=tc  ActiveDisplayYMinimum=-1578.7453878307324  ActiveDisplayYMaximum=1578.7340154658184  DataLoggingVariableName=ScopeData4
  dab current output/input modA : Scope  NumInputPorts=2
      settings: SampleTime=tc  ActiveDisplayYMinimum=-410.50779379600635  ActiveDisplayYMaximum=588.57119970360964  DataLoggingVariableName=ScopeData8
  dab outputs modA : Scope  NumInputPorts=2
      settings: SampleTime=tc  ActiveDisplayYMinimum=-911.87281827356537  ActiveDisplayYMaximum=678.26507696890121  DataLoggingVariableName=ScopeData6
  dab voltage input/output modA : Scope  NumInputPorts=2
      settings: SampleTime=tc  ActiveDisplayYMinimum=1151.9301233458582  ActiveDisplayYMaximum=1294.7889710686802  DataLoggingVariableName=ScopeData10
  dab_analysis : Scope  NumInputPorts=4
      settings: SampleTime=tc  ActiveDisplayYMinimum=-2819.8939411691067  ActiveDisplayYMaximum=1653.00985583068  DataLoggingVariableName=ScopeData14
  i0_transformer : Scope  NumInputPorts=2
      settings: SampleTime=tc  ActiveDisplayYMinimum=-1.8947806286936003E-13  ActiveDisplayYMaximum=1.8947806286936003E-13  DataLoggingVariableName=ScopeData11
  inverter_1_thermal_data : Scope  NumInputPorts=4
      settings: SampleTime=tc  ActiveDisplayYMinimum=-41.628226428892724  ActiveDisplayYMaximum=374.65403786003458
  inverter_2_thermal_data : Scope  NumInputPorts=4
      settings: SampleTime=tc  ActiveDisplayYMinimum=-51.964921296072347  ActiveDisplayYMaximum=467.68429166465125  DataLoggingVariableName=ScopeData9
  wires:
  [i1_dab_transformer_modA] -> dab_analysis/3  "i1_tr"
  [u1_dab_transformer_modA] -> dab_analysis/4  "u1_tr"
  [i2_dab_transformer_modA] -> dab_analysis/1  "i2_tr"
  [u2_dab_transformer_modA] -> dab_analysis/2  "u2_tr"
  [u10_dab_transformer_modA] -> i0_transformer/1
  [i2_dab0_transformer_modA] -> i0_transformer/2
  [inverter_2_dab_devices_modA] -> Bus Selector1/1
  Bus Selector1/1 -> inverter_2_thermal_data/1  "<mosfet_ploss_Q1>"
  Bus Selector1/2 -> inverter_2_thermal_data/2  "<mosfet_ploss_Q3>"
  Bus Selector1/3 -> inverter_2_thermal_data/3  "<mosfet_ploss_Q4>"
  Bus Selector1/4 -> inverter_2_thermal_data/4  "<mosfet_ploss_Q2>"
  Bus Selector/4 -> inverter_1_thermal_data/4  "<mosfet_ploss_Q2>"
  Bus Selector/3 -> inverter_1_thermal_data/3  "<mosfet_ploss_Q4>"
  Bus Selector/2 -> inverter_1_thermal_data/2  "<mosfet_ploss_Q3>"
  Bus Selector/1 -> inverter_1_thermal_data/1  "<mosfet_ploss_Q1>"
  [inverter_1_dab_devices_modA] -> Bus Selector/1
  [dab_current_output_modA] -> dab outputs modA/1  "dab_current_output_modA"
  [dab_voltage_output_modA] -> dab outputs modA/2  "dab_voltage_output_modA"
  [u1_dab_transformer_modA] -> dab TR u2/u1 modA/2  "u1_dab_transformer_modA"
  [u2_dab_transformer_modA] -> dab TR u2/u1 modA/1  "u2_dab_transformer_modA"
  [i1_dab_transformer_modA] -> dab TR i2/i1 modA/2  "i1_dab_transformer_modA"
  [i2_dab_transformer_modA] -> dab TR i2/i1 modA/1  "i2_dab_transformer_modA"
  [dab_current_input_modA] -> dab current output/input modA/2  "dab_current_input_modA"
  [dab_voltage_output_modA] -> dab voltage input/output modA/2  "dab_voltage_output_modA"
  [dab_current_output_modA] -> dab current output/input modA/1  "dab_current_output_modA"
  [dab_voltage_input_modA] -> dab voltage input/output modA/1  "dab_voltage_input_modA"

== system sst_three_phase_dab_three_levels_inv/dab_modB/dcdc_with_galvanic_isolation/single_phase_dab_transformer ==
  three_phase_hf_transformer : Subsystem
  threephase_vi_measures_stack : Subsystem
  threephase_vi_measures_stack1 : Subsystem
  u1 : PMIOPort  Side=Left
  v1 : PMIOPort  Port=2  Side=Left
  w1 : PMIOPort  Port=3  Side=Left
  u2 : PMIOPort  Port=4  Side=Right
  v2 : PMIOPort  Port=5  Side=Right
  w2 : PMIOPort  Port=6  Side=Right
  connections:
  threephase_vi_measures_stack1/RConn1 -- u2/RConn1
  w2/RConn1 -- threephase_vi_measures_stack1/RConn3
  v2/RConn1 -- threephase_vi_measures_stack1/RConn2
  w1/RConn1 -- threephase_vi_measures_stack/LConn3
  v1/RConn1 -- threephase_vi_measures_stack/LConn2
  u1/RConn1 -- threephase_vi_measures_stack/LConn1
  threephase_vi_measures_stack/RConn4 -- three_phase_hf_transformer/LConn4
  threephase_vi_measures_stack1/LConn4 -- three_phase_hf_transformer/RConn4
  threephase_vi_measures_stack1/LConn3 -- three_phase_hf_transformer/RConn3
  threephase_vi_measures_stack1/LConn2 -- three_phase_hf_transformer/RConn2
  threephase_vi_measures_stack1/LConn1 -- three_phase_hf_transformer/RConn1
  three_phase_hf_transformer/LConn3 -- threephase_vi_measures_stack/RConn3
  three_phase_hf_transformer/LConn2 -- threephase_vi_measures_stack/RConn2
  three_phase_hf_transformer/LConn1 -- threephase_vi_measures_stack/RConn1

== system sst_three_phase_dab_three_levels_inv/dab_modB/dcdc_with_galvanic_isolation/three_phase_inverter_1 ==
  gate_commands : Inport
  dclink_1 : Subsystem
  three_phase_inverter_1 : Subsystem
  u : PMIOPort  Side=Left
  v : PMIOPort  Port=2  Side=Left
  Udc(+) : PMIOPort  Port=3  Side=Right
  Udc(-) : PMIOPort  Port=4  Side=Right
  w : PMIOPort  Port=5  Side=Left
  wires:
  gate_commands/1 -> three_phase_inverter_1/1(gate_commands)
  connections:
  w/RConn1 -- three_phase_inverter_1/RConn3
  three_phase_inverter_1/LConn2 -- dclink_1/RConn2
  three_phase_inverter_1/RConn2 -- v/RConn1
  three_phase_inverter_1/RConn1 -- u/RConn1
  dclink_1/RConn1 -- three_phase_inverter_1/LConn1
  Udc(-)/RConn1 -- dclink_1/LConn2
  Udc(+)/RConn1 -- dclink_1/LConn1

== system sst_three_phase_dab_three_levels_inv/dab_modB/dcdc_with_galvanic_isolation/three_phase_inverter_2 ==
  gate_commands : Inport
  dclink_2 : Subsystem
  three_phase_inverter_2 : Subsystem
  u : PMIOPort  Side=Left
  v : PMIOPort  Port=2  Side=Left
  udc(+) : PMIOPort  Port=3  Side=Right
  udc(-) : PMIOPort  Port=4  Side=Right
  w : PMIOPort  Port=5  Side=Left
  wires:
  gate_commands/1 -> three_phase_inverter_2/1(gate_commands)
  connections:
  w/RConn1 -- three_phase_inverter_2/LConn3
  dclink_2/LConn2 -- three_phase_inverter_2/RConn2
  v/RConn1 -- three_phase_inverter_2/LConn2
  u/RConn1 -- three_phase_inverter_2/LConn1
  dclink_2/LConn1 -- three_phase_inverter_2/RConn1
  udc(-)/RConn1 -- dclink_2/RConn2
  udc(+)/RConn1 -- dclink_2/RConn1

== system sst_three_phase_dab_three_levels_inv/inverter_modA/single phase inverter control1/acquisition_and_scaling_current ==
  in : Inport
  1/Ti5 : Gain  Gain=1/Iac_FS  SaturateOnIntegerOverflow=on  OutDataTypeStr=Inherit: Same as input  ParamDataTypeStr=Inherit: Same as input
  out : Outport
  wires:
  in/1 -> 1/Ti5/1
  1/Ti5/1 -> out/1

== system sst_three_phase_dab_three_levels_inv/inverter_modA/single phase inverter control1/acquisition_and_scaling_dc_voltage ==
  in : Inport
  1/Ti3 : Gain  Gain=1/Vdc_FS  SaturateOnIntegerOverflow=on  OutDataTypeStr=Inherit: Same as input  ParamDataTypeStr=Inherit: Same as input
  out : Outport
  wires:
  in/1 -> 1/Ti3/1
  1/Ti3/1 -> out/1

== system sst_three_phase_dab_three_levels_inv/inverter_modA/single phase inverter control1/acquisition_and_scaling_voltage ==
  in : Inport
  1/Ti5 : Gain  Gain=1/Vac_FS  SaturateOnIntegerOverflow=on  OutDataTypeStr=Inherit: Same as input  ParamDataTypeStr=Inherit: Same as input
  out : Outport
  wires:
  in/1 -> 1/Ti5/1
  1/Ti5/1 -> out/1

== system sst_three_phase_dab_three_levels_inv/inverter_modA/single phase inverter control1/acquisition_and_scaling_voltage1 ==
  in : Inport
  1/Ti1 : Gain  Gain=1/Vac_FS  SaturateOnIntegerOverflow=on  OutDataTypeStr=Inherit: Same as input  ParamDataTypeStr=Inherit: Same as input
  1/Ti2 : Gain  Gain=1/n_modules  SaturateOnIntegerOverflow=on  OutDataTypeStr=Inherit: Same as input  ParamDataTypeStr=Inherit: Same as input
  out : Outport
  wires:
  in/1 -> 1/Ti2/1
  1/Ti1/1 -> out/1
  1/Ti2/1 -> 1/Ti1/1

== system sst_three_phase_dab_three_levels_inv/inverter_modA/single phase inverter control1/inverter_current_output_pu_reference ==
  Gain : Gain  Gain=-1
  Rate Limiter : RateLimiter  RisingSlewLimit=50  FallingSlewLimit=-50  SampleTimeMode=inherited
  Sum : Sum  Inputs=|++
  i_out_inverter_reference_step1 : Step  Time=0.05  After=iph_grid_pu_ref  SampleTime=0
  i_out_inverter_reference_step2 : Step  Commented=on  Time=0.25  After=-iph_grid_pu_ref  SampleTime=0
  inverter_current_output_pu_reference : Outport
  wires:
  Rate Limiter/1 -> Gain/1
  Sum/1 -> Rate Limiter/1
  i_out_inverter_reference_step1/1 -> Sum/1
  i_out_inverter_reference_step2/1 -> Sum/2
  Gain/1 -> inverter_current_output_pu_reference/1

== system sst_three_phase_dab_three_levels_inv/inverter_modA/single phase inverter control1/pwm modulator ==
  vout : Inport
  Constant : Constant  Value=0
  single_phase_three_levels_PWM_generator_with_global_TRGO : single_phase_three_levels_PWM_modulator/single_phase_three_levels_PWM_generator_with_global_TRGO  f=fPWM_INV  m_up=1  m_low=-1  dead_time=dead_time_INV  pos_cmd_gate=15  neg_cmd_gate=-10  polarity=1  tc=tc  double_sampling=1
  gate_cmds : Outport
  tag scope: TRGO_INV_1=global
  wires:
  vout/1 -> single_phase_three_levels_PWM_generator_with_global_TRGO/3
  [time_afe_module_1] -> single_phase_three_levels_PWM_generator_with_global_TRGO/1
  Constant/1 -> single_phase_three_levels_PWM_generator_with_global_TRGO/2
  single_phase_three_levels_PWM_generator_with_global_TRGO/2 -> gate_cmds/1
  single_phase_three_levels_PWM_generator_with_global_TRGO/1 -> [TRGO_INV_1]

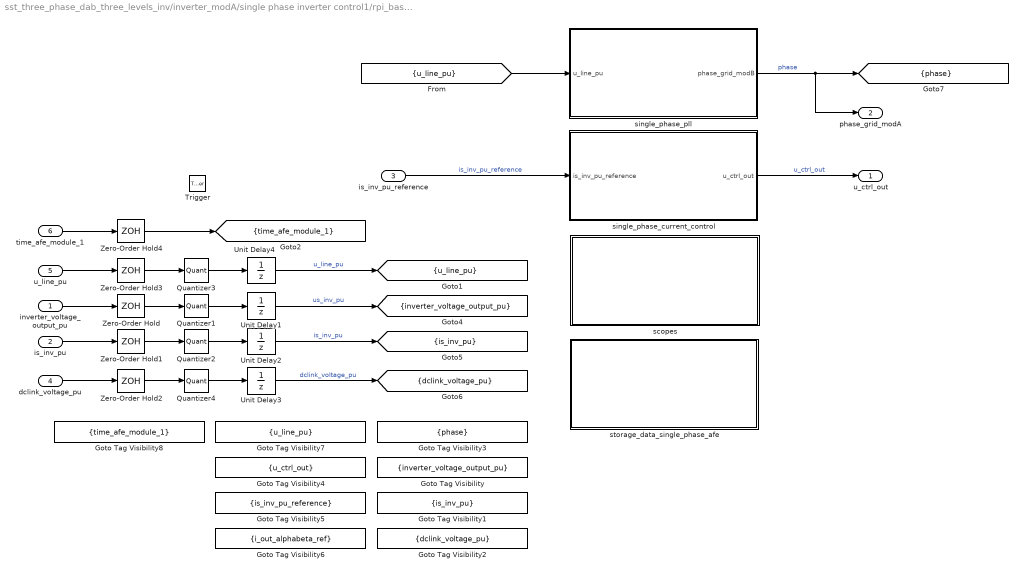
== system sst_three_phase_dab_three_levels_inv/inverter_modA/single phase inverter control1/rpi_based_single_phase_inverter_ctrl ==
  inverter_voltage_output_pu : Inport
  is_inv_pu : Inport  Port=2
  is_inv_pu_reference : Inport  Port=3
  dclink_voltage_pu : Inport  Port=4
  u_line_pu : Inport  Port=5
  time_afe_module_1 : Inport  Port=6
  Trigger : TriggerPort  VariantControl=(inherit)  PortDimensions=1
  Goto Tag Visibility : GotoTagVisibility  GotoTag=inverter_voltage_output_pu
  Goto Tag Visibility1 : GotoTagVisibility  GotoTag=is_inv_pu
  Goto Tag Visibility2 : GotoTagVisibility  GotoTag=dclink_voltage_pu
  Goto Tag Visibility3 : GotoTagVisibility  GotoTag=phase
  Goto Tag Visibility4 : GotoTagVisibility  GotoTag=u_ctrl_out
  Goto Tag Visibility5 : GotoTagVisibility  GotoTag=is_inv_pu_reference
  Goto Tag Visibility6 : GotoTagVisibility  GotoTag=i_out_alphabeta_ref
  Goto Tag Visibility7 : GotoTagVisibility  GotoTag=u_line_pu
  Goto Tag Visibility8 : GotoTagVisibility  GotoTag=time_afe_module_1
  Quantizer{1..4} (4 alike) : Quantizer  QuantizationInterval=adc12_quantization
  Unit Delay{1..4} (4 alike) : UnitDelay  SampleTime=-1  HasFrameUpgradeWarning=on
  Zero-Order Hold{,1..4} (5 alike) : ZeroOrderHold  SampleTime=-1
  scopes : Subsystem
  single_phase_current_control : Subsystem
  single_phase_pll : Subsystem
  storage_data_single_phase_afe : Subsystem
  u_ctrl_out : Outport
  phase_grid_modA : Outport  Port=2
  tag scope: dclink_voltage_pu=scoped, inverter_voltage_output_pu=scoped, is_inv_pu=scoped, phase=scoped, time_afe_module_1=scoped, u_line_pu=scoped
  wires:
  inverter_voltage_output_pu/1 -> Zero-Order Hold/1
  is_inv_pu/1 -> Zero-Order Hold1/1
  dclink_voltage_pu/1 -> Zero-Order Hold2/1
  Unit Delay1/1 -> [inverter_voltage_output_pu]  "us_inv_pu"
  Unit Delay2/1 -> [is_inv_pu]  "is_inv_pu"
  Unit Delay3/1 -> [dclink_voltage_pu]  "dclink_voltage_pu"
  is_inv_pu_reference/1 -> single_phase_current_control/1(is_inv_pu_reference)  "is_inv_pu_reference"
  single_phase_current_control/1(u_ctrl_out) -> u_ctrl_out/1  "u_ctrl_out"
  u_line_pu/1 -> Zero-Order Hold3/1
  Quantizer1/1 -> Unit Delay1/1
  Quantizer2/1 -> Unit Delay2/1
  Quantizer4/1 -> Unit Delay3/1
  Quantizer3/1 -> Unit Delay4/1
  single_phase_pll/1(phase_grid_modB) -> phase_grid_modA/1, [phase]  "phase"
  Zero-Order Hold/1 -> Quantizer1/1
  Zero-Order Hold1/1 -> Quantizer2/1
  Zero-Order Hold2/1 -> Quantizer4/1
  Unit Delay4/1 -> [u_line_pu]  "u_line_pu"
  [u_line_pu] -> single_phase_pll/1(u_line_pu)
  Zero-Order Hold3/1 -> Quantizer3/1
  time_afe_module_1/1 -> Zero-Order Hold4/1
  Zero-Order Hold4/1 -> [time_afe_module_1]
